simulink model "Simulation_trifasic_motor"  (R2025a)
settings: Solver=ode23tb  StartTime=0.0  StopTime=10  MaxStep=10e-6  RelTol=1e-4
libraries: spsControlledVoltageSourceLib x2, spsAsynchronousMachineSIUnitsLib x1, spsFourierLib x1, spsPowerLib x1, spspowerguiLib x1, spsVoltageMeasurementLib x1
settings Model: ExtModeTrigMode=oneshot  ExtModeArmWhenConnect=off  ExtModeAutoUpdateStatusClock=off  Creator=The MathWorks, Inc.  LastModifiedBy=tequi
settings SolverCC: AlgebraicLoopSolver=TrustRegion
settings DataIOCC: ExternalInput=[]  SaveFormat=Array  SaveOutput=off  ReturnWorkspaceOutputs=off  TimeSaveName=t  SignalLoggingName=sigsOut
settings OptimizationCC: BlockReduction=off  BooleanDataType=off  ExpressionDepthLimit=2147483647.0  InitFltsAndDblsToZero=on  EfficientMapNaN2IntZero=off  LifeSpan=inf
settings DebuggingCC: UnderspecifiedInitializationDetection=Classic  MergeDetectMultiDrivingBlocksExec=none  CheckExecutionContextPreStartOutputMsg=on  SignalResolutionControl=TryResolveAllWithWarning  MultiTaskDSMMsg=warning  MultiTaskCondExecSysMsg=none  SigSpecEnsureSampleTimeMsg=none  FcnCallInpInsideContextMsg=warning  UnconnectedLineMsg=warning  StateNameClashWarn=warning  SFUnexpectedBacktrackingDiag=warning  SFNoUnconditionalDefaultTransitionDiag=warning  SFExecutionAtInitializationDiag=none  ArithmeticOperatorsInVariantConditions=warning
settings HardwareCC: ProdBitPerPointer=32.0  ProdBitPerSizeT=32.0  ProdBitPerPtrDiffT=32.0  ProdLargestAtomicFloat=None  ProdIntDivRoundTo=Undefined  ProdEndianess=Unspecified  ProdWordSize=32.0  ProdHWDeviceType=32-bit Generic  TargetUnknown=on
settings ModelReferenceCC: EnableRefExpFcnMdlSchedulingChecks=on  PropagateSignalLabelsOutOfModel=off
settings SFSimCC: SimUseLocalCustomCode=off  CustomCodeUndefinedFunction=UseInterfaceOnly
settings RTWCC: RTWUseLocalCustomCode=off  GPUComputeCapability=3.5  DLArmComputeVersion=19.05
settings CodeAppCC: StateflowObjectComments=on
settings GRTTargetCC: TargetLangStandard=C89/C90 (ANSI)  CombineOutputUpdateFcns=off  GRTInterface=on
settings ConfigComp: CovMetricSettings=dw  CovSaveCumulativeToWorkspaceVar=on  CovSaveSingleToWorkspaceVar=on  CovExternalEMLEnable=off  CovSFcnEnable=off
settings SimscapeCC: SimscapeNormalizeSystem=off

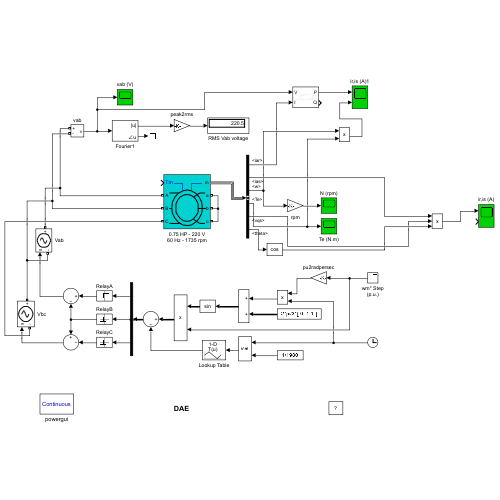
[thumbnail: Simulink's stored preview of the top-level diagram]
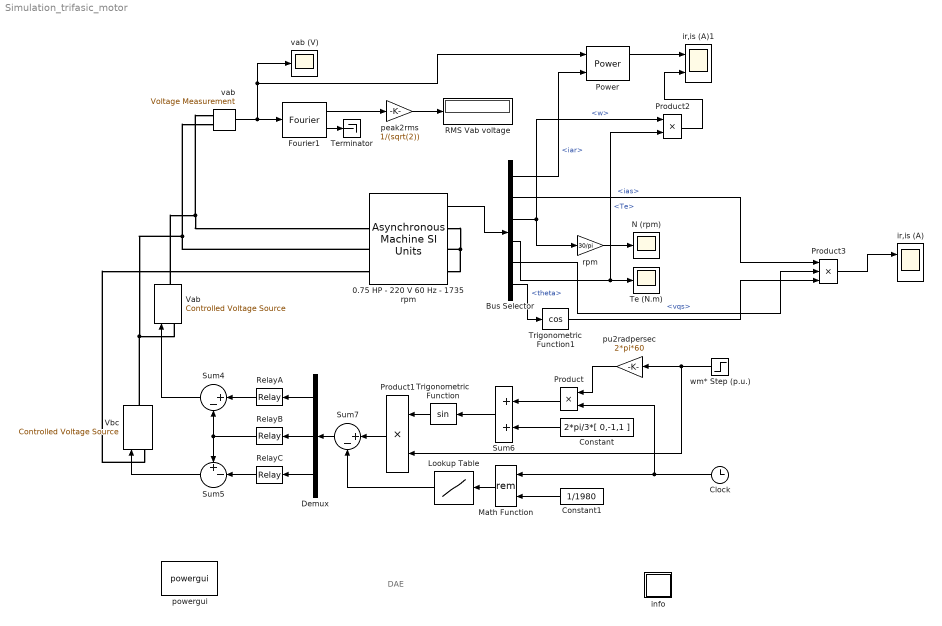
== system Simulation_trifasic_motor ==
  note: DAE
  0.75 HP - 220 V 60 Hz - 1735 rpm : spsAsynchronousMachineSIUnitsLib/Asynchronous Machine SI Units  RotorType=Wound  PresetModel=No  MechanicalLoad=Torque Tm  ShowDetailedParameters=on  ReferenceFrame=Stationary  Units=SI  MeasurementBus=on  NominalParameters=[ 0.75*746, 220, 60 ]  VoltageRatio=1  Stator="[ 0.435  2*2.0e-3 ]"  Rotor="[ 0.816  2.0e-3 ]"  Cage1=[ 0.022 0.226/377]  Cage2=[ 0.022 0.226/377]  Lm=69.31e-3  Mechanical="[ 0.089  0 2]"  PolePairs=2  InitialConditions="[ 1,0   0,0,0   0,0,0 ]"  SimulateSaturation=off  Saturation=[14.03593122, 27.81365428, 53.79336849, 72.68890987, 97.98006896, 148.6815601, 215.7428561, 302.9841135, 428.7778367 ; 230, 322, 414, 460, 506, 552, 598, 644, 690]  LoadFlowParameters=0  TsPowergui=0  TsBlock=-1  IterativeModel=Trapezoidal non iterative  IterativeDiscreteModel=Trapezoidal non iterative  Pmec=0
      settings: AttributesFormatString=\n
  Bus Selector : BusSelector  OutputSignals=iar,ias,w,Te,vqs,theta
  Clock : Clock
  Constant : Constant  Value=2*pi/3*[ 0,-1,1 ]
  Constant1 : Constant  Value=1/1980
  Demux : Demux  Outputs=3
      settings: DisplayOption=none
  Fourier1 : spsFourierLib/Fourier  Freq=60  n=1  InInit=[0, 0]  Ts=0
  Lookup Table : Lookup_n-D  NumberOfTableDimensions=1  BreakpointsForDimension1="[0 0.25  0.75  1] / 1980"  BreakpointsForDimension2=[0 571.55 685.8 800.15 914.4 1028.8 1143.1 1257.4 1371.7 1486 1600.3 1714.6 1828.9 1943.2 2057.5 2171.8 2286.1 2400.5 2514.7 2629.1 2743.3 2857.7 2971.9 3086.3 3200.5 3314.9 3429.2]  Table="[0  1  -1  0]"  InternalRulePriority=Speed  RndMeth=Simplest
  Math Function : Math  Operator=rem  SignedPower=on
  N (rpm) : Scope
      settings: ActiveDisplayYMinimum=1730.34512  ActiveDisplayYMaximum=1863.93216  DataLoggingSaveFormat=Array
  Power : spsPowerLib/Power  Freq=60  Vinit=[1, 0]  Iinit=[1, 0]  Ts=0
  Product : Product  InputSameDT=on  SaturateOnIntegerOverflow=on  OutDataTypeStr=Inherit: Same as first input
  Product1 : Product  InputSameDT=on  SaturateOnIntegerOverflow=on  OutDataTypeStr=Inherit: Same as first input
  Product2 : Product  InputSameDT=on  SaturateOnIntegerOverflow=on  OutDataTypeStr=Inherit: Same as first input
  Product3 : Product  Inputs=3  InputSameDT=on  SaturateOnIntegerOverflow=on  OutDataTypeStr=Inherit: Same as first input
  RMS Vab voltage : Display
      settings: Decimation=100
  RelayA : Relay  OnSwitchValue=0  OffSwitchValue=0  OnOutputValue=220*sqrt(2/3)  OffOutputValue=-220*sqrt(2/3)
  RelayB : Relay  OnSwitchValue=0  OffSwitchValue=0  OnOutputValue=220*sqrt(2/3)  OffOutputValue=-220*sqrt(2/3)
  RelayC : Relay  OnSwitchValue=0  OffSwitchValue=0  OnOutputValue=220*sqrt(2/3)  OffOutputValue=-220*sqrt(2/3)
  Sum4 : Sum  Inputs=|+-  InputSameDT=on  SaturateOnIntegerOverflow=on  OutDataTypeStr=Inherit: Same as first input
  Sum5 : Sum  Inputs=+-|  InputSameDT=on  SaturateOnIntegerOverflow=on  OutDataTypeStr=Inherit: Same as first input
  Sum6 : Sum  InputSameDT=on  SaturateOnIntegerOverflow=on  OutDataTypeStr=Inherit: Same as first input
  Sum7 : Sum  Inputs=|+-  InputSameDT=on  SaturateOnIntegerOverflow=on  OutDataTypeStr=Inherit: Same as first input
  Te (N.m) : Scope
      settings: ActiveDisplayYMinimum=-8.50353  ActiveDisplayYMaximum=10.06498  DataLoggingSaveFormat=Array
  Terminator : Terminator
  Trigonometric Function : Trigonometry
  Trigonometric Function1 : Trigonometry  Operator=cos
  Vab : spsControlledVoltageSourceLib/Controlled Voltage Source  Description=source block  Initialize=on  Source_Type=AC  Amplitude=0  Phase=0  Frequency=0  Measurements=None
      settings: AttributesFormatString=\n
  Vbc : spsControlledVoltageSourceLib/Controlled Voltage Source  Description=source block  Initialize=on  Source_Type=AC  Amplitude=0  Phase=0  Frequency=0  Measurements=None
      settings: AttributesFormatString=\n
  info : Subsystem
      settings: OpenFcn="showExample(\"simscapeelectricalsps/ThreePhaseASMExample\")"
      mask Display: disp('?')
  ir,is (A) : Scope  NumInputPorts=2
      settings: TimeSpan=1  ActiveDisplayYMinimum=-1193.6243343697502  ActiveDisplayYMaximum=1782.285663561875  DataLoggingSaveFormat=Array
  ir,is (A)1 : Scope  NumInputPorts=2
      settings: TimeSpan=1  ActiveDisplayYMinimum=-13058.8475  ActiveDisplayYMaximum=13510.47928  DataLoggingSaveFormat=Array
  peak2rms : Gain  Gain=1/(sqrt(2))  SaturateOnIntegerOverflow=on  OutDataTypeStr=Inherit: Same as input  ParamDataTypeStr=Inherit: Same as input
  powergui : spspowerguiLib/powergui  SimulationMode=Continuous  SampleTime=0  frequency=60  Iterations=50  frequencyindice=60  Pbase=100e6  ErrMax=1e-4  UnitsV=kV  UnitsW=MW  buscounter=0  FunctionMessages=off  echomessages=off  EnableUseOfTLC=off  CurrentSourceSwitches=off  DisableSnubberDevices=off  DisableRonSwitches=off  DisableVfSwitches=off  DisplayEquations=off  AutomaticDiscreteSolvers=off  SolverType=Tustin  Interpol=off  ExternalGateDelay=off  methode=off  Ts=0  x0status=blocks  SPID=on  SwTol=0  HookPort=off  NonlinearTolerance=1e-4  nMaxIteration=100  ContinueOnMaxIteration=off  RestoreLinks=warning  ResistiveCurrentMeasurement=off  Frange=[0:2:500]  Ylog=off  Xlog=on  ShowGrid=off  save=off  variable=ZData  structure=0  ZoomFFT=on  StartTime=0.0  cycles=1  DisplayStyle=1  fundamental=60  FreqAxis=off  MaxFrequency=1000  frequencyindicesteady=1  RmsSteady=1  display=off
  pu2radpersec : Gain  Gain=2*pi*60  SaturateOnIntegerOverflow=on  OutDataTypeStr=Inherit: Same as input  ParamDataTypeStr=Inherit: Same as input
  rpm : Gain  Gain=30/pi  SaturateOnIntegerOverflow=on  OutDataTypeStr=Inherit: Same as input  ParamDataTypeStr=Inherit: Same as input
  vab : spsVoltageMeasurementLib/Voltage Measurement  Tag=PoWeRsYsTeMmEaSuReMeNt  PhasorSimulation=off  OutputType=Magnitude  PSBequivalent=0
  vab (V) : Scope
      settings: ActiveDisplayYMinimum=-382.67931  ActiveDisplayYMaximum=369.08687  DataLoggingSaveFormat=Array
  wm* Step (p.u.) : Step  Time=0  SampleTime=0
  wires:
  RelayA/1 -> Sum4/1
  RelayC/1 -> Sum5/2
  RelayB/1 -> Sum5/1, Sum4/2
  Demux/2 -> RelayB/1
  Demux/3 -> RelayC/1
  Demux/1 -> RelayA/1
  Sum7/1 -> Demux/1
  pu2radpersec/1 -> Product/1
  Sum6/1 -> Trigonometric Function/1
  Trigonometric Function/1 -> Product1/1
  Product1/1 -> Sum7/1
  wm* Step (p.u.)/1 -> pu2radpersec/1, Product1/2
  Lookup Table/1 -> Sum7/2
  Clock/1 -> Math Function/1, Product/2
  Math Function/1 -> Lookup Table/1
  Constant1/1 -> Math Function/2
  Product/1 -> Sum6/1
  Constant/1 -> Sum6/2
  Fourier1/1 -> peak2rms/1
  Fourier1/2 -> Terminator/1
  Bus Selector/4 -> Product2/2, Te (N.m)/1  "<Te>"
  rpm/1 -> N (rpm)/1
  Sum4/1 -> Vab/1
  Sum5/1 -> Vbc/1
  vab/1 -> Fourier1/1, vab (V)/1, Power/1
  Bus Selector/1 -> Power/2  "<iar>"
  0.75 HP - 220 V 60 Hz - 1735 rpm/1 -> Bus Selector/1
  Bus Selector/3 -> rpm/1, Product2/1  "<w>"
  peak2rms/1 -> RMS Vab voltage/1
  Power/1 -> ir,is (A)1/1
  Product2/1 -> ir,is (A)1/2
  Bus Selector/6 -> Trigonometric Function1/1  "<theta>"
  Trigonometric Function1/1 -> Product3/3
  Bus Selector/2 -> Product3/1  "<ias>"
  Bus Selector/5 -> Product3/2  "<vqs>"
  Product3/1 -> ir,is (A)/1
  connections:
  Vbc/LConn1 -- 0.75 HP - 220 V 60 Hz - 1735 rpm/LConn3
  Vab/RConn1 -- vab/LConn1 -- 0.75 HP - 220 V 60 Hz - 1735 rpm/LConn1
  0.75 HP - 220 V 60 Hz - 1735 rpm/LConn2 -- Vab/LConn1 -- Vbc/RConn1 -- vab/LConn2
  0.75 HP - 220 V 60 Hz - 1735 rpm/RConn1 -- 0.75 HP - 220 V 60 Hz - 1735 rpm/RConn3 -- 0.75 HP - 220 V 60 Hz - 1735 rpm/RConn2

== system Simulation_trifasic_motor/info ==
